simulink model "double_cylinder_spring"  (R2024b)
settings: Solver=VariableStepAuto  StartTime=0.0  StopTime=10.0  RelTol=1e-3
values from neighbouring files (symbols this model uses):
  F = 2    [parameters.m]
  m1 = 1    [parameters.m]
  x1 = 0.2    [parameters.m]
  x2 = 0    [parameters.m]
undefined symbols (not defined in the file or in its folder): k, km
settings Model: Creator=kavin  LastModifiedBy=kavin

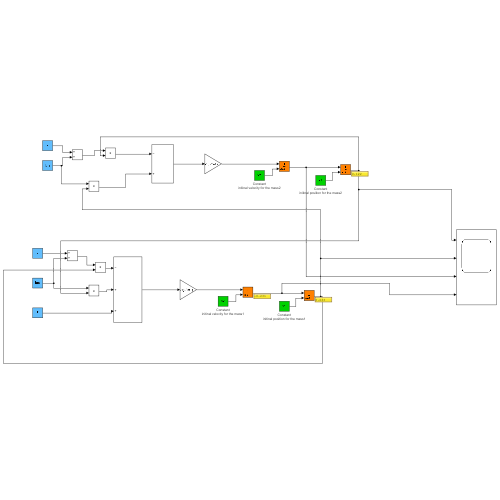
[thumbnail: Simulink's stored preview of the top-level diagram]
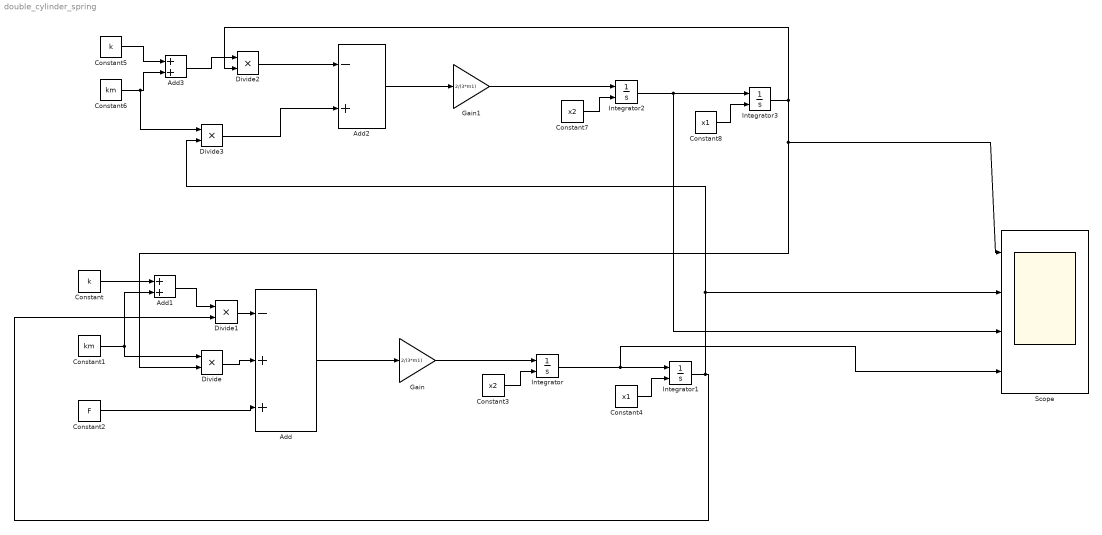
== system double_cylinder_spring ==
  Add : Sum  Inputs=-++
  Add1 : Sum
  Add2 : Sum  Inputs=-+
  Add3 : Sum
  Constant : Constant  Value=k
  Constant1 : Constant  Value=km
  Constant2 : Constant  Value=F
  Constant3 : Constant  Value=x2
      settings: AttributesFormatString=|
      | %<BlockType>
      | initinal velocity for the mass1
  Constant4 : Constant  Value=x1
      settings: AttributesFormatString=|
      | %<BlockType>
      | initinal position for the mass1
  Constant5 : Constant  Value=k
  Constant6 : Constant  Value=km
  Constant7 : Constant  Value=x2
      settings: AttributesFormatString=|
      | %<BlockType>
      | initinal velocity for the mass2
  Constant8 : Constant  Value=x1
      settings: AttributesFormatString=|
      | %<BlockType>
      | initinal position for the mass2
  Divide{,1..3} (4 alike) : Product  Inputs=**
  Gain : Gain  Gain=2/(3*m1)
  Gain1 : Gain  Gain=2/(3*m1)
  Integrator{,1..3} (4 alike) : Integrator  InitialConditionSource=external
  Scope : Scope  NumInputPorts=4
  wires:
  Constant1/1 -> Divide/1, Add1/2
  Constant/1 -> Add1/1
  Add1/1 -> Divide1/1
  Constant2/1 -> Add/3
  Add/1 -> Gain/1
  Gain/1 -> Integrator/1
  Constant3/1 -> Integrator/2
  Constant4/1 -> Integrator1/2
  Divide1/1 -> Add/1
  Integrator1/1 -> Scope/2, Divide3/2, Divide1/2
  Integrator2/1 -> Scope/3, Integrator3/1
  Constant8/1 -> Integrator3/2
  Constant7/1 -> Integrator2/2
  Gain1/1 -> Integrator2/1
  Add2/1 -> Gain1/1
  Divide2/1 -> Add2/1
  Constant5/1 -> Add3/1
  Constant6/1 -> Divide3/1, Add3/2
  Add3/1 -> Divide2/1
  Divide3/1 -> Add2/2
  Integrator3/1 -> Divide/2, Scope/1, Divide2/2
  Integrator/1 -> Scope/4, Integrator1/1
  Divide/1 -> Add/2
